simulink model "sf_test_vectors"  (Simulink 7.6)
settings: Solver=ode5  SolverMode=SingleTasking  StartTime=0.0  StopTime=30  RelTol=1e-3  AbsTol=1e-6
PreLoadFcn:
  | load sldemo_autotrans_data;
undefined symbols (not defined in the file or in its folder): converter_data, downtab, emap, Iei, sigbuilder_block, uptab, vehicledata
Description:
  | Modelling an Automatic Transmission Controller
  | 
  | In this example, we use Simulink to model an automotive drivetrain. We also use Stateflow to
  | model the automatic transmission control logic. In many systems, supervisory functions such as
  | changing modes or invoking new gain schedules must respond to events that may occur and
  | conditions that develop over time. You can use Stateflow to model such functionality as
  | shown in this example, where we use Stateflow to perform the function of gear selection in an
  | automatic transmission. This function is combined with the drivetrain dynamics in a natural
  | and intuitive manner by incorporating a Stateflow block in the Simulink block diagram.
  | 
  | The Stateflow block labeled shift_logic implements gear selection for the transmission. The
  | dashed lines indicate parallel (AND) states which keep track of the gear state and the state
  | of the gear selection process. The overall chart is executed as a discrete-time system. The
  | Stateflow diagram is shown below. The shift logic behavior can be observed during simulation by enabling animation in the
  | Stateflow debugger.
settings Model: Creator=The MathWorks Inc.  CovMetricSettings=dcmtr  ExtModeTrigMode=oneshot  ExtModeArmWhenConnect=off  ExtModeAutoUpdateStatusClock=off
settings SolverCC: InsertRTBMode=Auto
settings DataIOCC: LimitDataPoints=off  SaveOutput=off  SaveTime=off  SignalLoggingName=sigsOut
settings OptimizationCC: BlockReduction=off  BooleanDataType=off  InlineInvariantSignals=on  InitFltsAndDblsToZero=on
settings DebuggingCC: SaveWithParameterizedLinksMsg=none  CheckExecutionContextPreStartOutputMsg=on  CheckExecutionContextRuntimeOutputMsg=on  SignalResolutionControl=TryResolveAllWithWarning  SolverPrmCheckMsg=none  MultiTaskDSMMsg=warning  MultiTaskCondExecSysMsg=none  SigSpecEnsureSampleTimeMsg=none  IntegerOverflowMsg=none  StrictBusMsg=None
settings HardwareCC: TargetUnknown=on
settings SFSimCC: SFSimEcho=off  SimParseCustomCode=off
settings RTWCC: IncludeERTFirstTime=on
settings GRTTargetCC: TargetFcnLib=ansi_tfl_tmw.mat

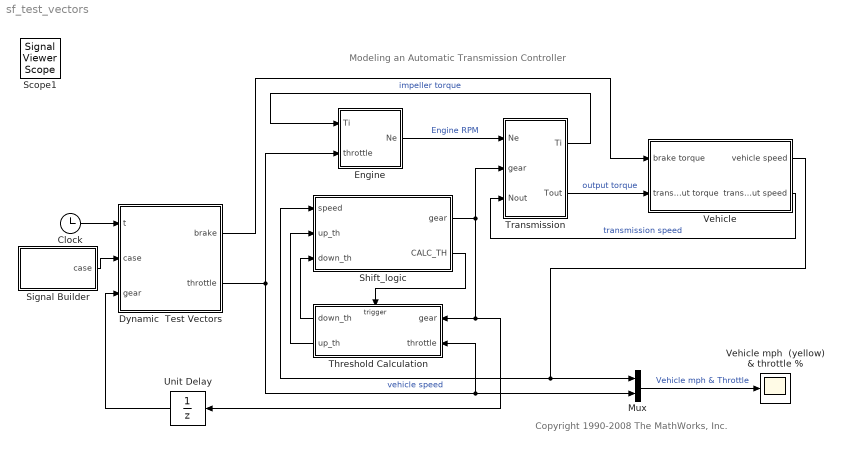
== system sf_test_vectors ==
  note: Modeling an Automatic Transmission Controller
  note: Copyright 1990-2008 The MathWorks, Inc.
  Clock : Clock
  Dynamic  Test Vectors : Stateflow chart  TreatAsAtomicUnit=on
  Engine : Subsystem
  Mux : Mux  Inputs=2
  Shift_logic : Stateflow chart  TreatAsAtomicUnit=on
  Signal Builder : Subsystem  Tag=STV Subsys  LoadFcn=sigbuilder_block('load');  StartFcn=sigbuilder_block('start');  StopFcn=sigbuilder_block('stop');  ClipboardFcn=sigbuilder_block('clipboard');  mask(Sigbuilder block){}
      mask help: Sigbuilder GUI
      mask init:
      | if ~strcmp(get_param(bdroot(gcbh),'SimulationStatus'),'stopped') tuvar = sigbuilder_block('maskInit'); end
      settings: CopyFcn=sigbuilder_block('copy');  DeleteFcn=sigbuilder_block('delete');  ModelCloseFcn=sigbuilder_block('modelClose');  PreSaveFcn=sigbuilder_block('preSave');  NameChangeFcn=sigbuilder_block('namechange');  OpenFcn=sigbuilder_block('open',[47.2 128 550.4 398.4 ]);  CloseFcn=sigbuilder_block('close');
      mask Display: plot(0,0,100,100,[10,10,40,40,10],[80,20,20,80,80],[40,10],[50,50], [40,27,10],[65,72,56],[40,25,25,10],[28,28,43,43]);
  Threshold Calculation : Subsystem  TreatAsAtomicUnit=on
  Transmission : Subsystem
  Unit Delay : UnitDelay
  Vehicle : Subsystem  mask(vehicle model){Rfd=vehicledata(1), rload0=vehicledata(2), rload2=vehicledata(3), Rw=vehicledata(4), Iv=vehicledata(5), N20=vehicledata(6)/vehicledata(4)*vehicledata(1)}
      mask prompts: Rfd "final drive ratio"; rload0 "drag friction at wheels"; rload2 "aerodynamic drag"; Rw "wheel radius"; Iv "vehicle inertia"; N20 "initial transmission output speed"
      mask help: vehicle dynamics: torque input from trans., outputs are input speed (transmission output) and vehicle speed
      mask Display: image(imread([matlabroot,'/toolbox/simulink/simdemos/automotive/html/NSX_3Colors.jpg']))
  Vehicle mph  (yellow) & throttle % : Scope
      settings: TickLabels=on  TimeRange=30  YMin=0  YMax=150  DataFormat=Array
  Scope1 : SignalViewerScope  IOType=viewer  RefreshTime=0.035000
      settings: TimeRange=30  YMin=1000  YMax=5000
  wires:
  Transmission/1(Ti) -> Engine/1(Ti)  "impeller torque"
  Dynamic  Test Vectors/2(throttle) -> Engine/2(throttle), Mux/2, Threshold Calculation/2(throttle)
  Engine/1(Ne) -> Transmission/1(Ne)  "Engine RPM"
  Transmission/2(Tout) -> Vehicle/2(transmission output torque)  "output torque"
  Vehicle/2(transmission output speed) -> Transmission/3(Nout)  "transmission speed"
  Threshold Calculation/1(down_th) -> Shift_logic/3(down_th)
  Threshold Calculation/2(up_th) -> Shift_logic/2(up_th)
  Shift_logic/1(gear) -> Transmission/2(gear), Threshold Calculation/1(gear), Unit Delay/1
  Shift_logic/2(CALC_TH) -> Threshold Calculation/Trigger
  Vehicle/1(vehicle speed) -> Mux/1, Shift_logic/1(speed)  "vehicle speed"
  Mux/1 -> Vehicle mph  (yellow) & throttle %/1  "Vehicle mph & Throttle"
  Dynamic  Test Vectors/1(brake) -> Vehicle/1(brake torque)
  Clock/1 -> Dynamic  Test Vectors/1(t)
  Signal Builder/1(case) -> Dynamic  Test Vectors/2(case)
  Unit Delay/1 -> Dynamic  Test Vectors/3(gear)

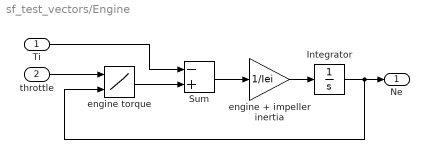
== system sf_test_vectors/Engine ==
  Ti : Inport
  throttle : Inport  Port=2
  Integrator : Integrator  InitialCondition=1000  LimitOutput=on  UpperSaturationLimit=6000  LowerSaturationLimit=600  ZeroCross=off
  Sum : Sum  Inputs=-+  SaturateOnIntegerOverflow=on  InputSameDT=on  OutDataTypeStr=Inherit: Same as first input
  engine torque : Lookup2D  RowIndex=thvec  ColumnIndex=nevec  Table=emap  InputSameDT=on
  engine + impeller inertia : Gain  Gain=1/Iei  SaturateOnIntegerOverflow=on  OutDataTypeStr=Inherit: Same as input  ParamDataTypeStr=Inherit: Same as input
  Ne : Outport  InitialOutput=0
  wires:
  Ti/1 -> Sum/1
  throttle/1 -> engine torque/1
  Integrator/1 -> engine torque/2, Ne/1
  Sum/1 -> engine + impeller inertia/1
  engine + impeller inertia/1 -> Integrator/1
  engine torque/1 -> Sum/2

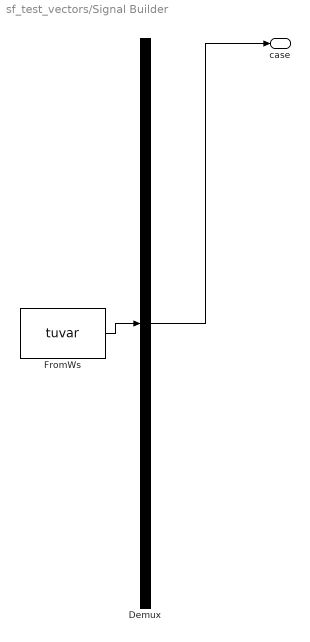
== system sf_test_vectors/Signal Builder ==
  Demux : Demux  Tag=STV Demux  Outputs=1
  FromWs : FromWorkspace  Tag=STV FromWs  VariableName=tuvar  SampleTime=0  SigBuilderData=DataTag0  VnvData=DataTag1
      SigBuilderData=|
      | common.afterFinalStr = 'Extrapolate'
      | common.sampleTime = 0
      | dataSet(1).timeRange = [0 10]
      | dataSet(1).name = 'Passing Maneuver'
      | dataSet(2).timeRange = [0 10]
      | dataSet(2).name = 'Gradual Acceleration'
      | dataSet(3).timeRange = [0 10]
      | dataSet(3).name = 'Hard Braking'
      | dataSet(4).timeRange = [0 10]
      | dataSet(4).name = 'Coasting'
      | sbobj.Name = 'Signal Builder'
      | sbobj.Groups(1).Name = 'Passing Maneuver'
      | sbobj.Groups(1).Signals.Name = 'case'
      | sbobj.Groups(1).Signals.XData = [0 10]
      | sbobj.Groups(1).Signals.YData = [1 1]
      | sbobj.Groups(2).Name = 'Gradual Acceleration'
      | sbobj.Groups(2).Signals.Name = 'case'
      | sbobj.Groups(2).Signals.XData = [0 10]
      | sbobj.Groups(2).Signals.YData = [2 2]
      | sbobj.Groups(3).Name = 'Hard Braking'
      | sbobj.Groups(3).Signals.Name = 'case'
      | sbobj.Groups(3).Signals.XData = [0 10]
      | sbobj.Groups(3).Signals.YData = [3 3]
      | sbobj.Groups(4).Name = 'Coasting'
      | sbobj.Groups(4).Signals.Name = 'case'
      | sbobj.Groups(4).Signals.XData = [0 10]
      | sbobj.Groups(4).Signals.YData = [4 4]
  case : Outport  Tag=STV Outport
  wires:
  Demux/1 -> case/1
  FromWs/1 -> Demux/1

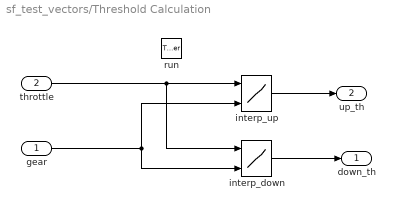
== system sf_test_vectors/Threshold Calculation ==
  gear : Inport
  throttle : Inport  Port=2
  run : TriggerPort  TriggerType=function-call  ZeroCross=off
  interp_down : Lookup2D  RowIndex=downth  ColumnIndex=[1:4]  Table=downtab  InputSameDT=on
  interp_up : Lookup2D  RowIndex=upth  ColumnIndex=[1:4]  Table=uptab  InputSameDT=on
  down_th : Outport
  up_th : Outport  Port=2
  wires:
  interp_up/1 -> up_th/1
  interp_down/1 -> down_th/1
  throttle/1 -> interp_up/1, interp_down/1
  gear/1 -> interp_up/2, interp_down/2

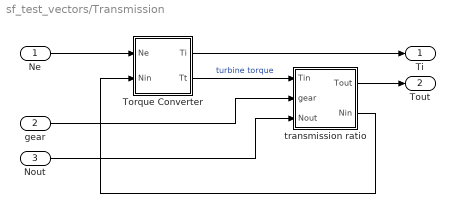
== system sf_test_vectors/Transmission ==
  Ne : Inport
  gear : Inport  Port=2
  Nout : Inport  Port=3
  Torque Converter : Subsystem  mask(torque converter){speedratio=converter_data(:,1), Kfactor=converter_data(:,2), Torkratio=converter_data(:,3)}
      mask prompts: speedratio "speed ratio"; Kfactor "K factor"; Torkratio "torque ratio"
      mask help: torque converter
      mask Help: Torque converter input and output torques are computed as a function of the input and output speeds
      mask Display: plot([cos([90:10:450]*pi/180),.63*cos([90:10:450]*pi/180),.63*cos([90:10:240]*pi/180),cos([240:10:300]*pi/180),.63*cos([300]*pi/180)],[sin([90:10:450]*pi/180),.63*sin([90:10:450]*pi/180)+.1,.63*sin([90:10:240]*pi/180)+.1,sin([240:10:300]*pi/180),.63*sin([300]*pi/180)+.1])
  transmission ratio : Subsystem
  Ti : Outport  InitialOutput=0
  Tout : Outport  Port=2  InitialOutput=0
  wires:
  transmission ratio/1(Tout) -> Tout/1
  Torque Converter/1(Ti) -> Ti/1
  Nout/1 -> transmission ratio/3(Nout)
  gear/1 -> transmission ratio/2(gear)
  Ne/1 -> Torque Converter/1(Ne)
  transmission ratio/2(Nin) -> Torque Converter/2(Nin)
  Torque Converter/2(Tt) -> transmission ratio/1(Tin)  "turbine torque"

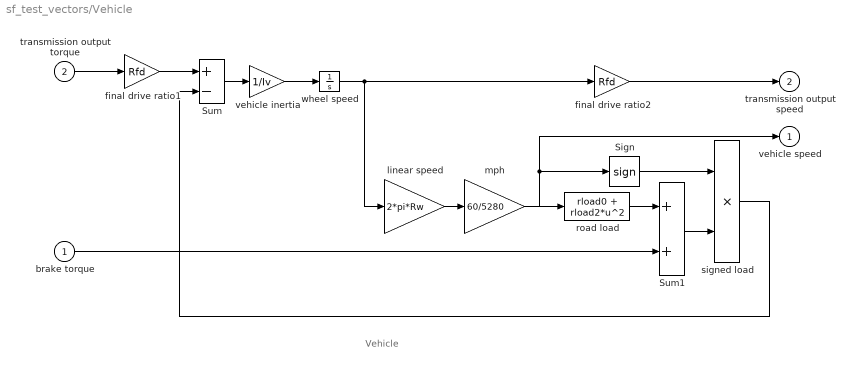
== system sf_test_vectors/Vehicle ==
  note: Vehicle
  brake torque : Inport
  transmission output torque : Inport  Port=2
  Sign : Signum
  Sum : Sum  Inputs=+-  SaturateOnIntegerOverflow=on  InputSameDT=on  OutDataTypeStr=Inherit: Same as first input
  Sum1 : Sum  SaturateOnIntegerOverflow=on  InputSameDT=on  OutDataTypeStr=Inherit: Same as first input
  final drive ratio1 : Gain  Gain=Rfd  SaturateOnIntegerOverflow=on  OutDataTypeStr=Inherit: Same as input  ParamDataTypeStr=Inherit: Same as input
  final drive ratio2 : Gain  Gain=Rfd  SaturateOnIntegerOverflow=on  OutDataTypeStr=Inherit: Same as input  ParamDataTypeStr=Inherit: Same as input
  linear speed : Gain  Gain=2*pi*Rw  SaturateOnIntegerOverflow=on  OutDataTypeStr=Inherit: Same as input  ParamDataTypeStr=Inherit: Same as input
  mph : Gain  Gain=60/5280  SaturateOnIntegerOverflow=on  OutDataTypeStr=Inherit: Same as input  ParamDataTypeStr=Inherit: Same as input
  road load : Fcn  Expr=rload0 + rload2*u^2
  signed load : Product  SaturateOnIntegerOverflow=on  InputSameDT=on  OutDataTypeStr=Inherit: Same as first input
  vehicle inertia : Gain  Gain=1/Iv  SaturateOnIntegerOverflow=on  OutDataTypeStr=Inherit: Same as input  ParamDataTypeStr=Inherit: Same as input
  wheel speed : Integrator  InitialCondition=N20/Rfd  ZeroCross=off
  vehicle speed : Outport  InitialOutput=0
  transmission output speed : Outport  Port=2  InitialOutput=0
  wires:
  final drive ratio2/1 -> transmission output speed/1
  brake torque/1 -> Sum1/2
  Sum1/1 -> signed load/2
  road load/1 -> Sum1/1
  Sign/1 -> signed load/1
  signed load/1 -> Sum/2
  transmission output torque/1 -> final drive ratio1/1
  vehicle inertia/1 -> wheel speed/1
  Sum/1 -> vehicle inertia/1
  mph/1 -> vehicle speed/1, Sign/1, road load/1
  linear speed/1 -> mph/1
  wheel speed/1 -> linear speed/1, final drive ratio2/1
  final drive ratio1/1 -> Sum/1

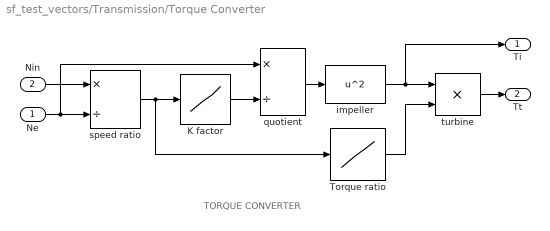
== system sf_test_vectors/Transmission/Torque Converter ==
  note: TORQUE CONVERTER
  Ne : Inport
  Nin : Inport  Port=2
  K factor : Lookup  InputValues=speedratio  Table=Kfactor  SaturateOnIntegerOverflow=on
  Torque ratio : Lookup  InputValues=speedratio  Table=Torkratio  SaturateOnIntegerOverflow=on
  impeller : Fcn  Expr=u^2
  quotient : Product  Inputs=*/  SaturateOnIntegerOverflow=on  InputSameDT=on  OutDataTypeStr=Inherit: Same as first input
  speed ratio : Product  Inputs=*/  SaturateOnIntegerOverflow=on  InputSameDT=on  OutDataTypeStr=Inherit: Same as first input
  turbine : Product  SaturateOnIntegerOverflow=on  InputSameDT=on  OutDataTypeStr=Inherit: Same as first input
  Ti : Outport  InitialOutput=0
  Tt : Outport  Port=2  InitialOutput=0
  wires:
  Torque ratio/1 -> turbine/2
  quotient/1 -> impeller/1
  K factor/1 -> quotient/2
  speed ratio/1 -> Torque ratio/1, K factor/1
  impeller/1 -> turbine/1, Ti/1
  turbine/1 -> Tt/1
  Ne/1 -> speed ratio/2, quotient/1
  Nin/1 -> speed ratio/1

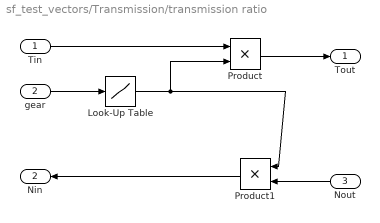
== system sf_test_vectors/Transmission/transmission ratio ==
  Tin : Inport
  gear : Inport  Port=2
  Nout : Inport  Port=3
  Look-Up Table : Lookup  InputValues=[1 2 3 4]  Table=[2.393 1.450 1.000 0.677]  SaturateOnIntegerOverflow=on
  Product : Product  SaturateOnIntegerOverflow=on  InputSameDT=on  OutDataTypeStr=Inherit: Same as first input
  Product1 : Product  SaturateOnIntegerOverflow=on  InputSameDT=on  OutDataTypeStr=Inherit: Same as first input
  Tout : Outport  InitialOutput=0
  Nin : Outport  Port=2  InitialOutput=0
  wires:
  Look-Up Table/1 -> Product1/1, Product/2
  Nout/1 -> Product1/2
  Product1/1 -> Nin/1
  Product/1 -> Tout/1
  Tin/1 -> Product/1
  gear/1 -> Look-Up Table/1

== stateflow chart Shift_logic ==
  settings: updateMethod=DISCRETE  sampleTime=0.04
  state gear_state [parallel]
    settings: executionOrder=1
    state fourth
      entry: gear = 4;
    state second
      entry: gear = 2;
    state third
      entry: gear = 3;
    state first
      entry: gear = 1;
    third -> fourth [order 1] : UP
    second -> third [order 1] : UP
    first -> second : UP
    (default) -> first
    fourth -> third : DOWN
    third -> second [order 2] : DOWN
    second -> first [order 2] : DOWN
  state selection_state [parallel]
    during: CALC_TH;
    settings: executionOrder=2
    state downshifting
    state upshifting
    state steady_state
    (default) -> steady_state
    steady_state -> upshifting [order 1] : [speed > up_th]
    steady_state -> downshifting [order 2] : [speed < down_th]
    upshifting -> steady_state [order 2] : [speed < up_th]
    downshifting -> steady_state [order 2] : [speed > down_th]
    downshifting -> steady_state [order 1] : after(TWAIT,tick)
        | [speed <= down_th]
        | {gear_state.DOWN}
    upshifting -> steady_state [order 1] : after(TWAIT,tick)
        | [speed >= up_th]
        | {gear_state.UP}
  data: speed input double; gear output uint8 [1..4] =1; TWAIT parameter uint8; up_th input double; down_th input double
  events: DOWN local EITHER_EDGE_EVENT; UP local EITHER_EDGE_EVENT; CALC_TH output FUNCTION_CALL_EVENT

== stateflow chart Dynamic Test Vectors ==
  state Coasting
    state Throttle [parallel]
      settings: executionOrder=2
      state A
        throttle=80;
      state B
        throttle=1;
      (default) -> Coasting.Throttle.A
      Coasting.Throttle.A -> Coasting.Throttle.B : [gear==4]
    state Brake [parallel]
      settings: executionOrder=1
      state A
        brake=0;
      (default) -> Coasting.Brake.A
  state HardBraking
    state Brake [parallel]
      settings: executionOrder=1
      state A
        brake=0;
      state B
        brake=325;
      (default) -> HardBraking.Brake.A
      HardBraking.Brake.A -> HardBraking.Brake.B : [t==10]
    state Throttle [parallel]
      settings: executionOrder=2
      state A
        throttle=50;
      state B
        throttle=1;
      (default) -> HardBraking.Throttle.A
      HardBraking.Throttle.A -> HardBraking.Throttle.B : [gear==3]
  state PassingManeuver
    state Throttle [parallel]
      settings: executionOrder=2
      state A
        du:throttle=(-4/3)*t+60;
      state B
        du:throttle=(-8/7)*(t-15)+100;
      (default) -> PassingManeuver.Throttle.A
      PassingManeuver.Throttle.A -> PassingManeuver.Throttle.B : [t==15]
    state Brake [parallel]
      settings: executionOrder=1
      state A
        brake=0;
      (default) -> PassingManeuver.Brake.A
  state GradualAcceleration
    state Throttle [parallel]
      settings: executionOrder=2
      state A
        du: throttle=(1/5)*t+14;
      (default) -> GradualAcceleration.Throttle.A
    state Brake [parallel]
      settings: executionOrder=1
      state A
        brake=0;
      (default) -> GradualAcceleration.Brake.A
  (default) -> PassingManeuver [order 1] : [case == 1]
  (default) -> Coasting [order 4]
  (default) -> GradualAcceleration [order 2] : [case==2]
  (default) -> HardBraking [order 3] : [case==3]
  data: t input double; brake output double; throttle output double; case input double; gear input double
